simulink library "Lib_Solve_DataOut_TMATS_new"  (R2015a)
settings: Solver=ode45  StartTime=0.0  StopTime=10.0  RelTol=1e-3
undefined symbols (not defined in the file): stripchar_TMATS
Description:
  | Thomas Modules
settings Model: CovSFcnEnable=off  Creator=jwchapm2  LastModifiedBy=jwhitfie
settings OptimizationCC: ExpressionDepthLimit=2147483647
settings DebuggingCC: UnderspecifiedInitializationDetection=Classic  MergeDetectMultiDrivingBlocksExec=none  SolverPrmCheckMsg=warning  StateNameClashWarn=warning

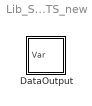
== system Lib_Solve_DataOut_TMATS_new ==
  DataOutput : Subsystem  mask(T-MATS: Data Output Library Block){FVar_M=strcat(stripchar_TMATS(gcb),'.bin')}
      mask prompts: FVar_M "FVar_M - File name for Variable Output"
      mask help: This Block saves the input variable to a file at each time step. Note, this will overwrite the previous value.
      mask init:
      | FVar_M = char(FVar_M);
      mask Help: web(which('Solver_TMATS_DOut.html'),'-helpbrowser')

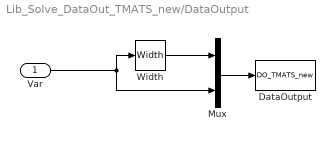
== system Lib_Solve_DataOut_TMATS_new/DataOutput ==
  Var : Inport
  DataOutput : S-Function  FunctionName=DO_TMATS_new  Parameters=FVar_M
  Mux : Mux  Inputs=2
  Width : Width
  wires:
  Var/1 -> Mux/2, Width/1
  Width/1 -> Mux/1
  Mux/1 -> DataOutput/1
